simulink model "HW2_2"  (R2018a)
settings: Solver=VariableStepAuto  StartTime=0.0  StopTime=10.0  RelTol=1e-3
undefined symbols (not defined in the file): B, J, K
settings Model: Creator=User  LastModifiedBy=User

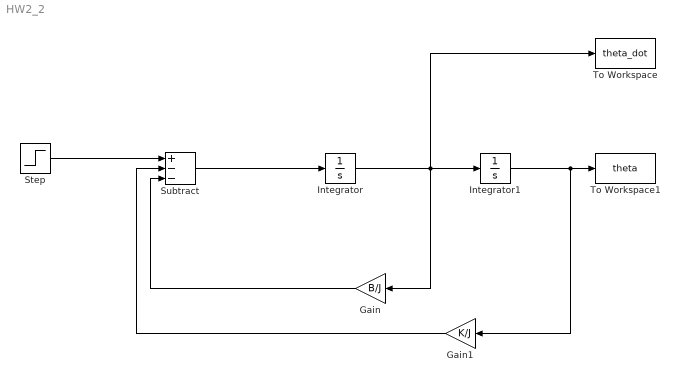
== system HW2_2 ==
  Gain : Gain  Gain=B/J
  Gain1 : Gain  Gain=K/J
  Integrator : Integrator
  Integrator1 : Integrator  InitialCondition=.175
  Step : Step  SampleTime=0
  Subtract : Sum  Inputs=+--
  To Workspace : ToWorkspace  VariableName=theta_dot  SaveFormat=Timeseries  SampleTime=-1
  To Workspace1 : ToWorkspace  VariableName=theta  SaveFormat=Timeseries  SampleTime=-1
  wires:
  Gain/1 -> Subtract/3
  Gain1/1 -> Subtract/2
  Integrator/1 -> To Workspace/1, Gain/1, Integrator1/1
  Subtract/1 -> Integrator/1
  Integrator1/1 -> To Workspace1/1, Gain1/1
  Step/1 -> Subtract/1
